simulink model "validacao_v1"  (R2018b)
settings: Solver=VariableStepAuto  StartTime=0.0  StopTime=1  RelTol=1e-3
libraries: simulink x1
settings Model: Creator=bernardo  LastModifiedBy=bernardo

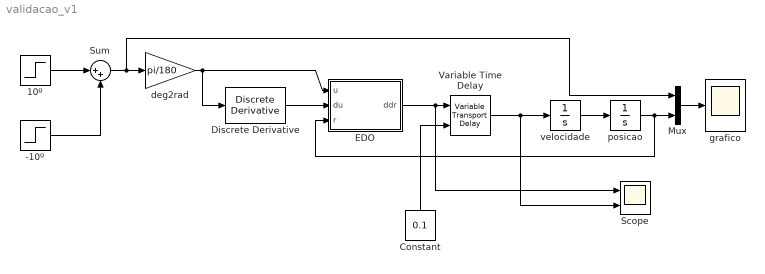
== system validacao_v1 ==
  -10º : Step  Time=10  After=10  SampleTime=0
  10º : Step  Time=5  Before=10  After=-10  SampleTime=0
  Constant : Constant  Value=0.1
  Discrete Derivative : simulink/Discrete/Discrete Derivative  gainval=1.0  ICPrevScaledInput=0.0  OutMin=[]  OutMax=[]  OutDataType=fixdt(1, 16)  OutScaling=2^-10  DoSatur=off
  EDO : MATLAB Function  TreatAsAtomicUnit=on
  Mux : Mux  Inputs=2
  Scope : Scope  NumInputPorts=2
  Sum : Sum  Inputs=|++
  Variable Time Delay : VariableTransportDelay  MaximumDelay=10
  deg2rad : Gain  Gain=pi/180
  grafico : Scope
  posicao : Integrator
  velocidade : Integrator
  wires:
  EDO/1(ddr) -> Scope/1, Variable Time Delay/1
  velocidade/1 -> posicao/1
  posicao/1 -> Mux/2, EDO/3(r)
  10º/1 -> Sum/1
  Discrete Derivative/1 -> EDO/2(du)
  deg2rad/1 -> Discrete Derivative/1, EDO/1(u)
  Mux/1 -> grafico/1
  Sum/1 -> Mux/1, deg2rad/1
  -10º/1 -> Sum/2
  Constant/1 -> Variable Time Delay/2
  Variable Time Delay/1 -> Scope/2, velocidade/1

== matlab function validacao_v1/EDO ==
  data: u input; ddr output; du input; r input
function ddr = fcn(u,du,r)
g = 981;              %%% cm/s²
d = 10.15;            %%% cm
L = 40;               %%% cm

mB = 3e-3;            %%% kg
R  = 2;               %%% cm
JB = 2*mB*R^2/3;      %%% kg*cm^2
a = mB + JB/R^2;
b = mB*d^2/L^2;
c = mB*g*d/L;

ddr = (b*du^2*r - c*sin(u))/a;
